simulink model "Flowchart9"  (Simulink 6.0)
settings: Solver=FixedStepDiscrete  StartTime=0.0  StopTime=10.0  RelTol=1e-3
settings Model: Creator=scaife  LastModifiedBy=scaife  ExtModeAutoUpdateStatusClock=off

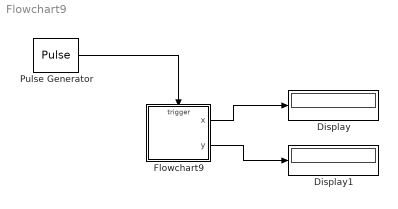
== system Flowchart9 ==
  Display : Display
  Display1 : Display
  Flowchart9 : Stateflow chart
  Pulse Generator : DiscretePulseGenerator
  wires:
  Flowchart9/1(x) -> Display/1
  Flowchart9/2(y) -> Display1/1
  Pulse Generator/1 -> Flowchart9/Trigger

== stateflow chart Flowchart9 ==
  state TOP [parallel]
    state A
      A -> (junction 6) : {x++}
    state B
      B -> (junction 7) : {y++}
    A -> B : E
    B -> A : E
    (default) -> A
  data: x output int32; y output int32
  events: E input EITHER_EDGE_EVENT
